simulink model "EulerAnglesFromAngularVelocity"  (R2021a)
settings: Solver=FixedStepAuto  StartTime=0.0  StopTime=200  RelTol=1e-3  EnableMultiTasking=on
undefined symbols (not defined in the file): DiscIntNeverNeededParam
libraries: arduinosensorlib x1
settings Model: SILPILModeSetting=veronly  ExtModeTrigDuration=2  Creator=Alireza  LastModifiedBy=admin
settings SolverCC: AlgebraicLoopSolver=TrustRegion
settings OptimizationCC: EnhancedBackFolding=on  PassReuseOutputArgsAs=Individual arguments  ZeroExternalMemoryAtStartup=off  ZeroInternalMemoryAtStartup=off  MaxStackSize=64  OptimizeBlockOrder=speed  DifferentSizesBufferReuse=on  OptimizationCustomize=off  EfficientTunableParamExpr=on
settings DebuggingCC: ParameterTunabilityLossMsg=error  SFMachineParentedDataDiag=warning  ArithmeticOperatorsInVariantConditions=warning
settings HardwareCC: ProdBitPerPointer=32  ProdBitPerSizeT=32  ProdBitPerPtrDiffT=32  ProdLargestAtomicInteger=Long  ProdLargestAtomicFloat=Double  ProdWordSize=32  ProdHWDeviceType=ARM Compatible->ARM Cortex
settings SFSimCC: MATLABDynamicMemAlloc=off  CustomCodeUndefinedFunction=UseInterfaceOnly
settings RTWCC: SystemTargetFile=ert.tlc  HardwareBoard=Arduino Due  TemplateMakefile=ert_default_tmf  Toolchain=Arduino ARM  BuildConfiguration=Faster Runs
settings CodeAppCC: ForceParamTrailComments=on  IgnoreCustomStorageClasses=off  OperatorAnnotations=on  SimulinkDataObjDesc=on  SFDataObjDesc=on  InsertBlockDesc=on
settings ERTTargetCC: SupportContinuousTime=on  SupportVariableSizeSignals=on  ExtModeTransport=3  ExtModeStaticAlloc=on  ExtModeStaticAllocSize=24576  ExtModeMexFile=ext_xcp  ExtModeIntrfLevel=Level2 - Open

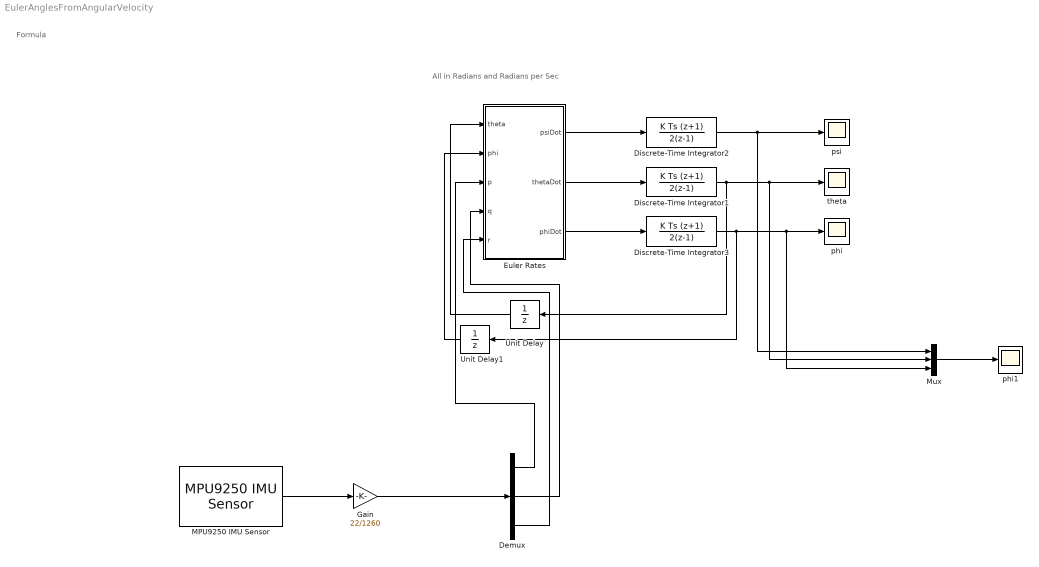
== system EulerAnglesFromAngularVelocity ==
  note: Formula
  note: All in Radians and Radians per Sec
  Demux : Demux  Outputs=3
  Discrete-Time Integrator1 : DiscreteIntegrator  IntegratorMethod=Integration: Trapezoidal  SampleTime=-1  ICPrevOutput=DiscIntNeverNeededParam  ICPrevScaledInput=DiscIntNeverNeededParam
  Discrete-Time Integrator2 : DiscreteIntegrator  IntegratorMethod=Integration: Trapezoidal  SampleTime=-1  ICPrevOutput=DiscIntNeverNeededParam  ICPrevScaledInput=DiscIntNeverNeededParam
  Discrete-Time Integrator3 : DiscreteIntegrator  IntegratorMethod=Integration: Trapezoidal  SampleTime=-1  ICPrevOutput=DiscIntNeverNeededParam  ICPrevScaledInput=DiscIntNeverNeededParam
  Euler Rates : Subsystem
  Gain : Gain  Gain=22/1260
  MPU9250 IMU Sensor : arduinosensorlib/MPU9250 IMU Sensor  SlaveAddress=0x68  Accel=off  AngularRate=on  Ak8963Field=off  Temperature=off  Status=off  EulerAngles=off  Quat=off  AccelRange=2G  Acceldlpf=218.1 Hz  GyroRange=250 dps  Gyrodlpf=250 Hz  DmpOdr=200 Hz  SampleTime=-1
      settings: SourceProductBaseCode=ARDUINO
  Mux : Mux  Inputs=3
  Unit Delay : UnitDelay  SampleTime=-1  HasFrameUpgradeWarning=on
  Unit Delay1 : UnitDelay  SampleTime=-1  HasFrameUpgradeWarning=on
  phi : Scope
  phi1 : Scope
  psi : Scope
  theta : Scope
  wires:
  Euler Rates/2(thetaDot) -> Discrete-Time Integrator1/1
  Unit Delay1/1 -> Euler Rates/2(phi)
  Unit Delay/1 -> Euler Rates/1(theta)
  Euler Rates/3(phiDot) -> Discrete-Time Integrator3/1
  Euler Rates/1(psiDot) -> Discrete-Time Integrator2/1
  Discrete-Time Integrator3/1 -> Unit Delay1/1, Mux/3, phi/1
  Discrete-Time Integrator1/1 -> Mux/2, theta/1, Unit Delay/1
  Discrete-Time Integrator2/1 -> Mux/1, psi/1
  Demux/1 -> Euler Rates/3(p)
  Demux/2 -> Euler Rates/4(q)
  Demux/3 -> Euler Rates/5(r)
  MPU9250 IMU Sensor/1 -> Gain/1
  Gain/1 -> Demux/1
  Mux/1 -> phi1/1

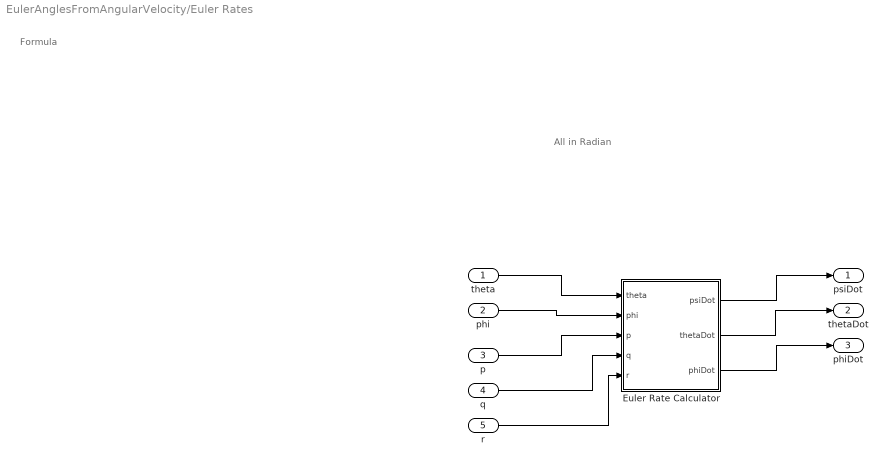
== system EulerAnglesFromAngularVelocity/Euler Rates ==
  note: All in Radian
  note: Formula
  theta : Inport
  phi : Inport  Port=2
  p : Inport  Port=3
  q : Inport  Port=4
  r : Inport  Port=5
  Euler Rate Calculator : MATLAB Function  TreatAsAtomicUnit=on
  psiDot : Outport
  thetaDot : Outport  Port=2
  phiDot : Outport  Port=3
  wires:
  phi/1 -> Euler Rate Calculator/2(phi)
  theta/1 -> Euler Rate Calculator/1(theta)
  p/1 -> Euler Rate Calculator/3(p)
  q/1 -> Euler Rate Calculator/4(q)
  r/1 -> Euler Rate Calculator/5(r)
  Euler Rate Calculator/1(psiDot) -> psiDot/1
  Euler Rate Calculator/2(thetaDot) -> thetaDot/1
  Euler Rate Calculator/3(phiDot) -> phiDot/1

== matlab function EulerAnglesFromAngularVelocity/Euler Rates/Euler Rate Calculator ==
  data: theta input; psiDot output; phi input; p input; q input; r input; thetaDot output; phiDot output
function [psiDot,thetaDot,phiDot] = fcn(theta,phi,p,q,r)

psiDot =  sin(phi)/cos(theta)*q + cos(phi)/cos(theta)*r;
thetaDot = cos(phi)*q - sin(phi)*r;
phiDot = p + sin(phi)*tan(theta)*q + cos(phi)*tan(theta)*r;
end
